simulink model "add"  (R2023a)
settings: Solver=VariableStepAuto  StartTime=0.0  StopTime=6  RelTol=1e-3
settings Model: Creator=levsi  LastModifiedBy=levsi

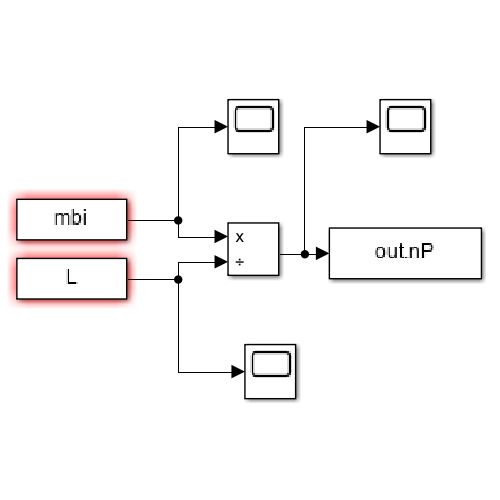
[thumbnail: Simulink's stored preview of the top-level diagram]
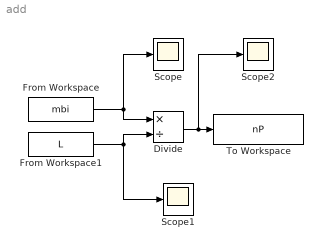
== system add ==
  Divide : Product  Inputs=*/
  From Workspace : FromWorkspace  VariableName=mbi  Interpolate=off  OutputAfterFinalValue=Setting to zero
  From Workspace1 : FromWorkspace  VariableName=L  Interpolate=off  OutputAfterFinalValue=Setting to zero
  Scope : Scope
  Scope1 : Scope
  Scope2 : Scope
  To Workspace : ToWorkspace  VariableName=nP  SaveFormat=Timeseries  SampleTime=0.001
  wires:
  From Workspace/1 -> Scope/1, Divide/1
  From Workspace1/1 -> Scope1/1, Divide/2
  Divide/1 -> Scope2/1, To Workspace/1
